simulink model "Simulink_model"  (R2022b)
settings: Solver=VariableStepAuto  StartTime=0.0  StopTime=10.0  RelTol=1e-3
values from neighbouring files (symbols this model uses):
  A = [0 1 0 ... (first row only)    [UnitVectorContoller.m]
  B = [zeros(2,1); 1/L0]    [UnitVectorContoller.m]
  Lrc = Leq + inv(S*B)*Caphi*S    [UnitVectorContoller.m]
  S = [M 1]    [UnitVectorContoller.m]
settings Model: Creator=henrr  LastModifiedBy=henrr

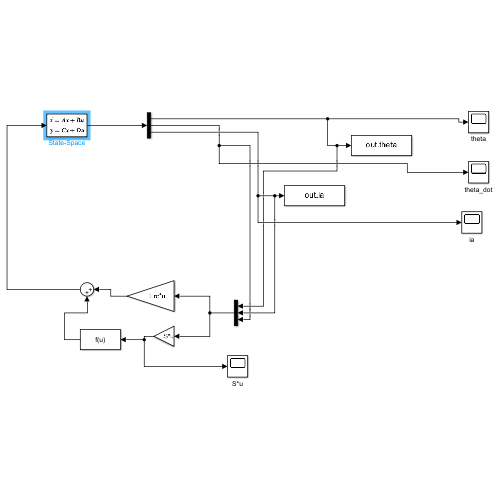
[thumbnail: Simulink's stored preview of the top-level diagram]
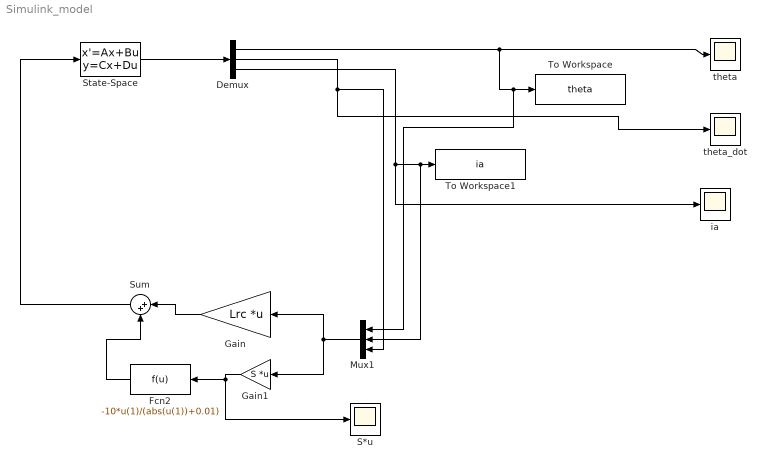
== system Simulink_model ==
  Demux : Demux  Outputs=3
  Fcn2 : Fcn  Expr=-10*u(1)/(abs(u(1))+0.01)
  Gain : Gain  Gain=Lrc  Multiplication=Matrix(K*u)
  Gain1 : Gain  Gain=S  Multiplication=Matrix(K*u)
  Mux1 : Mux  Inputs=3
  S*u : Scope
  State-Space : StateSpace  A=A  B=B  C=eye(3)  D=[0;0;0]  InitialCondition=[5;0;0]  ParameterTunability=Unconstrained
  Sum : Sum  Inputs=|++
  To Workspace : ToWorkspace  VariableName=theta  SaveFormat=Timeseries  SampleTime=-1
  To Workspace1 : ToWorkspace  VariableName=ia  SaveFormat=Timeseries  SampleTime=-1
  ia : Scope
  theta : Scope
  theta_dot : Scope
  wires:
  Demux/2 -> theta_dot/1, Mux1/3
  Demux/3 -> ia/1, Mux1/2, To Workspace1/1
  Demux/1 -> Mux1/1, To Workspace/1, theta/1
  Mux1/1 -> Gain1/1, Gain/1
  Gain/1 -> Sum/1
  Gain1/1 -> Fcn2/1, S*u/1
  Sum/1 -> State-Space/1
  State-Space/1 -> Demux/1
  Fcn2/1 -> Sum/2
